simulink model "LampToggler"  (Simulink 7.1)
settings: Solver=ode45  StartTime=0.0  StopTime=inf  RelTol=1e-3
libraries: simulink x1
settings Model: Creator=Meisel  LastModifiedBy=Meisel

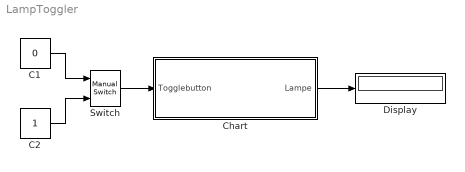
== system LampToggler ==
  C1 : Constant  Value=0  OutDataType=sfix(16)  OutScaling=2^0
  C2 : Constant  OutDataType=sfix(16)  OutScaling=2^0
  Chart : Stateflow chart
  Display : Display
  Switch : simulink/Signal Routing/Manual Switch  SystemSampleTime=-1  sw=1  action=0  varsize=off
  wires:
  C1/1 -> Switch/1
  C2/1 -> Switch/2
  Switch/1 -> Chart/1(Togglebutton)
  Chart/1(Lampe) -> Display/1

== stateflow chart Chart ==
  state Lampe_an
    entry: Lampe = 1
  state Lampe_aus
    entry: Lampe = 0
  state BtnOn_a
  state BtnOn_b
  (default) -> Lampe_an
  Lampe_aus -> BtnOn_b : [Togglebutton == 1]
  BtnOn_b -> Lampe_an : [Togglebutton == 0]
  Lampe_an -> BtnOn_a : [Togglebutton==1]
  BtnOn_a -> Lampe_aus : [Togglebutton == 0]
  data: Togglebutton input double; Lampe output double
